simulink model "cube0_mpcpd_ref_ls"  (R2022b)
settings: Solver=VariableStepAuto  StartTime=0.0  StopTime=3000  RelTol=1e-3  AbsTol=1e-3
settings Model: Creator=Abhijit  LastModifiedBy=abhij
settings SolverCC: AutoScaleAbsTol=off  AlgebraicLoopSolver=TrustRegion  MaxZcPerStep=1
settings DebuggingCC: UnconnectedInputMsg=warning  UnconnectedOutputMsg=warning  UnconnectedLineMsg=warning  SymbolicDimsDataTypeCodeGenerationDiagnostic=none  SFMachineParentedDataDiag=warning
settings ModelReferenceCC: EnableRefExpFcnMdlSchedulingChecks=on
settings SFSimCC: CustomCodeUndefinedFunction=UseInterfaceOnly
settings RTWCC: DLArmComputeVersion=19.05
settings SimscapeCC: SimscapeLogType=all  SimscapeLogSimulationStatistics=on  SimscapeLogDataHistory=10000

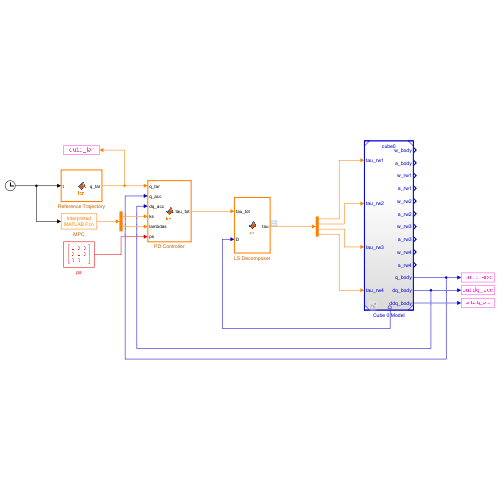
[thumbnail: Simulink's stored preview of the top-level diagram]
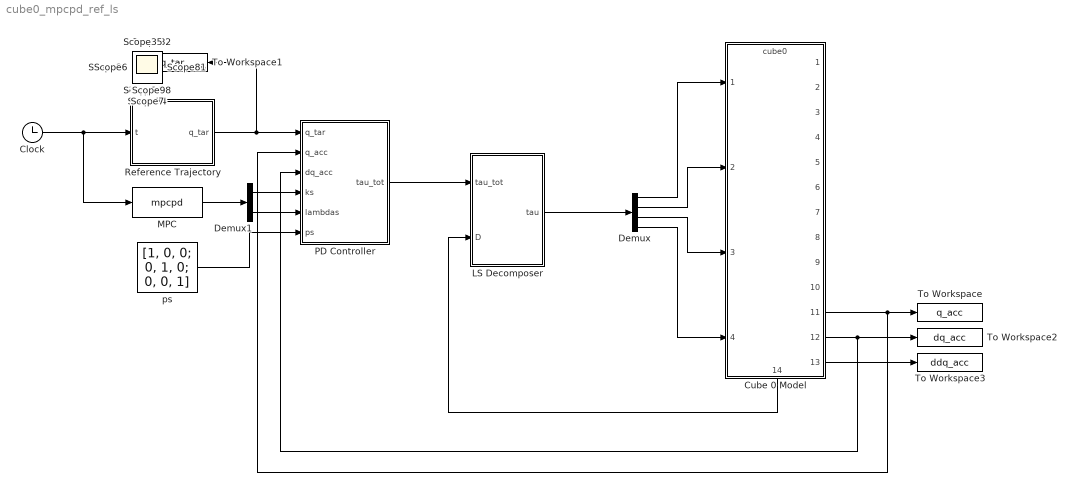
== system cube0_mpcpd_ref_ls ==
  Clock : Clock
  Cube 0 Model : ModelReference  ModelNameDialog=cube0.slx  SimulationMode=Normal  ModelReferenceVersion=1.8
      settings: PortSchema="{\"entries\":[{\"content\":{\"sides\":[{\"content\":{\"connectorIds\":[\"In1\",\"In2\",\"In3\",\"In4\"]},\"type\":\"ConnectorPlacement.EquallySpacedRectSide\",\"uuid\":\"8e9d2764-0c8c-4b35-a6b5-330d2d8aade7\"},{\"content\":{\"connectorIds\":[\"Out1\",\"Out2\",\"Out3\",\"Out4\",\"Out5\",\"Out6\",\"Out7\",\"Out8\",\"Out9\",\"Out10\",\"Out11\",\"Out12\",\"Out13\"],\"side\":\"RIGHT\"},\"type\":\"ConnectorPlacement.EquallySpacedRectSide\",\"uuid\":\"d11583f7-9081-4803-9c4e-bf58094124c2\"},{\"content\":{\"connectorIds\":[],\"side\":\"TOP\"},\"type\":\"ConnectorPlacement.EquallySpacedRectSide\",\"uuid\":\"f987c09c-5813-428e-a812-016ca0940eea\"},{\"content\":{\"connectorIds\":[\"Out14\"],\"side\":\"BOTTOM\"},\"type\":\"ConnectorPlacement.EquallySpacedRectSide\",\"uuid\":\"56fa612c-373e-46c3-86f2-ebb8be87bff3\"}]},\"type\":\"ConnectorPlacement.EquallySpacedConnector\",\"uuid\":\"9c548295-d181-4ae3-baad-4641f0a6e641\"}],\"packageUris\":[\"http://schema.mathworks.com/mf0/Connector/R2020b\"],\"version\":\"1.0\"}"
  Demux : Demux
  Demux1 : Demux  Outputs=2
  LS Decomposer : MATLAB Function  TreatAsAtomicUnit=on
  MPC : MATLABFcn  MATLABFcn=mpcpd  OutputDimensions=6
  PD Controller : MATLAB Function  TreatAsAtomicUnit=on
  Reference Trajectory : MATLAB Function  TreatAsAtomicUnit=on
  To Workspace : ToWorkspace  VariableName=q_acc  SaveFormat=Timeseries  SampleTime=-1
  To Workspace1 : ToWorkspace  VariableName=q_tar  SaveFormat=Timeseries  SampleTime=-1
  To Workspace2 : ToWorkspace  VariableName=dq_acc  SaveFormat=Timeseries  SampleTime=-1
  To Workspace3 : ToWorkspace  VariableName=ddq_acc  SaveFormat=Timeseries  SampleTime=-1
  ps : Constant  Value=[1, 0, 0; 0, 1, 0; 0, 0, 1]
  Scope{,1..35} (36 alike) : Scope
  wires:
  Clock/1 -> MPC/1, Reference Trajectory/1(t)
  Demux1/2 -> PD Controller/5(lambdas)
  Demux1/1 -> PD Controller/4(ks)
  ps/1 -> PD Controller/6(ps)
  Reference Trajectory/1(q_tar) -> To Workspace1/1, PD Controller/1(q_tar)
  Cube 0 Model/13 -> To Workspace3/1
  Cube 0 Model/12 -> To Workspace2/1, PD Controller/3(dq_acc)
  Cube 0 Model/11 -> To Workspace/1, PD Controller/2(q_acc)
  LS Decomposer/1(tau) -> Demux/1
  Demux/1 -> Cube 0 Model/1
  Demux/2 -> Cube 0 Model/2
  Demux/3 -> Cube 0 Model/3
  Demux/4 -> Cube 0 Model/4
  Cube 0 Model/14 -> LS Decomposer/2(D)
  PD Controller/1(tau_tot) -> LS Decomposer/1(tau_tot)
  MPC/1 -> Demux1/1

== matlab function cube0_mpcpd_ref_ls/PD Controller ==
  data: tau_tot output; q_tar input; q_acc input; dq_acc input; ks input; lambdas input; ps input
function tau_tot = fcn(q_tar, q_acc, dq_acc, ks, lambdas, ps)
    tau_tot = pdcontroller(q_tar, q_acc, dq_acc, ks, lambdas, ps);

== matlab function cube0_mpcpd_ref_ls/Reference Trajectory ==
  settings: updateMethod=CONTINUOUS
  data: t input; q_tar output
function q_tar = fcn(t)
     q_tar = refpath(t, 1);
end

== matlab function cube0_mpcpd_ref_ls/LS Decomposer ==
  data: tau_tot input; tau output; D input
function tau = fcn(tau_tot, D)
    tau = lsdecomp(tau_tot, D);
end
